simulink model "Wall_Model_Version_1_2"  (R2018a)
settings: Solver=ode3  StartTime=0.0  StopTime=Duration  FixedStep=Ts  RelTol=1e-3  EnableMultiTasking=on
InitFcn:
  | Ts=1;
  | Duration=36000;
  | %% Coefficients of Rs and Cs
  | y1 = 0.5
  | x1 = 0.33;
  | y2 = 0.5;
  | x2 = 0.33;
  | x3 = 0.33;
  | 
  | y3 = 0.5
  | x4 = 0.33;
  | y4 = 0.5;
  | x5 = 0.33;
  | x6 = 0.33;
  | 
  | y5 = 0.5
  | x7 = 0.33;
  | y6 = 0.5;
  | x8 = 0.33;
  | x9 = 0.33;
  | 
  | y7 = 0.5
  | x10 = 0.33;
  | y8 = 0.5;
  | x11 = 0.33;
  | x12= 0.33;
  | 
  | y9 = 0.5
  | x13 = 0.33;
  | y10 = 0.5;
  | x14 = 0.33;
  | x15 = 0.33;
  | 
  | y11 = 0.5
  | x16 = 0.33;
  | y12 = 0.5;
  | x17 = 0.33;
  | x18 = 0.33;
  | 
  | T1_initial_front=28;
  | T2_initial_front=27;
  | 
  | T1_initial_left=28;
  | T2_initial_left=27;
  | 
  | T1_initial_right=28;
  | T2_initial_right=27;
  | 
  | T1_initial_back=28;
  | T2_initial_back=27;
  | 
  | T1_initial_roof=28;
  | T2_initial_roof=27;
  | 
  | T1_initial_floor=28;
  | T2_initial_floor=27;
  | 
  | %% Resistance and Capacitance of front Wall
  | Rth1 = 1/0.8; % Common building brick conductivity = 0.8
  | Cth1 = 1000; % average thermal capcitance
  | 
  | %% Resistance and Capacitance of left Wall
  | Rth2 = 1/0.8; % Common building brick conductivity = 0.8
  | Cth2 = 1000; % average thermal capcitance
  | 
  | %% Resistance and Capacitance of right Wall
  | Rth3 = 1/0.8; % Common building brick conductivity = 0.8
  | Cth3 = 1000; % average thermal capcitance
  | 
  | %% Resistance and Capacitance of back Wall
  | Rth4 = 1/0.8; % Common building brick conductivity = 0.8
  | Cth4 = 1000; % average thermal capcitance
  | 
  | %% Resistance and Capacitance of roof Wall
  | Rth5 = 1/0.8; % Common building brick conductivity = 0.8
  | Cth5 = 1000; % average thermal capcitance
  | 
  | %% Resistance and Capacitance of floor Wall
  | Rth6 = 1/0.8; % Common building brick conductivity = 0.8
  | Cth6 = 1000; % average thermal capcitance
libraries: powerlib x66, simulink x1
settings Model: Creator=elekkr  LastModifiedBy=e0154145
settings DataIOCC: LimitDataPoints=on  SaveFormat=Array
settings OptimizationCC: LifeSpan=inf
settings DebuggingCC: UnconnectedInputMsg=none  UnconnectedOutputMsg=none  UnconnectedLineMsg=none  SFUnexpectedBacktrackingDiag=warning  SFNoUnconditionalDefaultTransitionDiag=warning  SFExecutionAtInitializationDiag=none
settings HardwareCC: ProdBitPerPointer=32  ProdBitPerSizeT=32  ProdBitPerPtrDiffT=32  ProdLargestAtomicFloat=None  ProdIntDivRoundTo=Undefined  ProdEndianess=Unspecified  ProdWordSize=32  ProdHWDeviceType=32-bit Generic
settings ModelReferenceCC: PropagateSignalLabelsOutOfModel=off
settings CodeAppCC: StateflowObjectComments=on
settings GRTTargetCC: TargetLangStandard=C89/C90 (ANSI)  GeneratePreprocessorConditionals=Disable all
settings ConfigComp: CovMetricSettings=dw  CovHtmlReporting=on  CovSaveCumulativeToWorkspaceVar=on  CovSaveSingleToWorkspaceVar=on  CovExternalEMLEnable=off
settings SimscapeCC: SimscapeNormalizeSystem=off

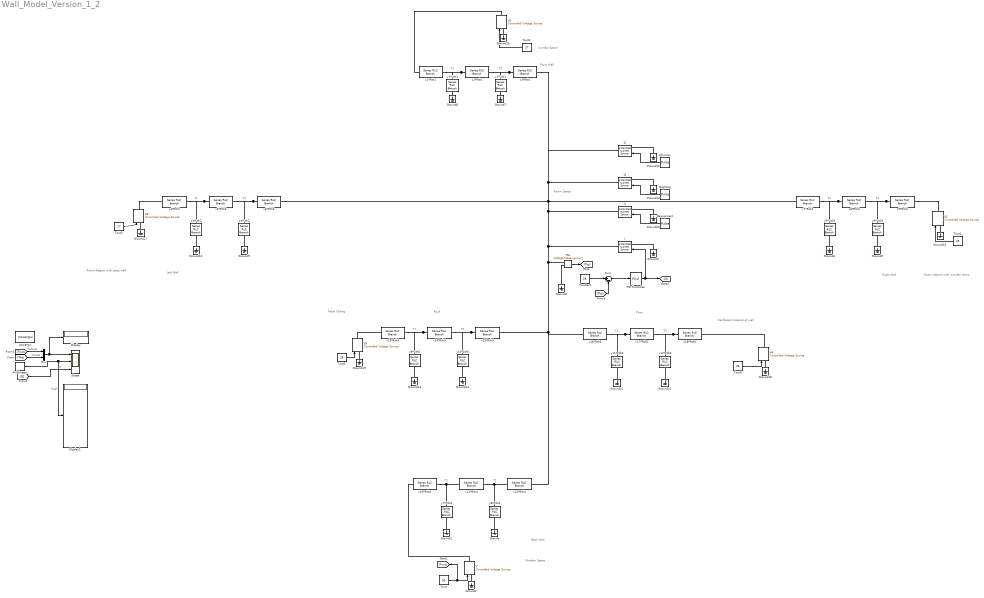
== system Wall_Model_Version_1_2 ==
  note: T1
  note: T2
  note: Back Wall
  note: Room Space
  note: Outdoor Space
  note: T1
  note: T2
  note: T1
  note: T2
  note: T1
  note: T2
  note: T2
  note: T1
  note: T1
  note: T2
  note: Right Wall
  note: Front Wall
  note: Left Wall
  note: Floor
  note: Roof
  note: Room Adjacnt with glass wall
  note: Corridpr Space
  note: Room Adjacnt with wooden doors
  note: Cardboard material of wall
  note: False Ceiling
  Constant : Constant  Value=28
  Display : Display
  Display1 : Display
  Ground{,1..22} (23 alike) : powerlib/Elements/Ground  LConnTagsString=a
  I{,1..3} (4 alike) : powerlib/Electrical Sources/Controlled Current Source  Initialize=on  Source_Type=AC  Amplitude=0  Phase=0  Frequency=0  Measurements=None
  Multimeter : powerlib/Measurements/Multimeter  PhasorSimulation=off  OutputType=Complex  sel=[1 2 3 4 5 6 7 8 9 10 11 12]  L=12  Gain=[1 1 1 1 1 1 1 1 1 1 1 1]  yselected={'Ub: y7*Cth4','Ub: y5*Cth3','Ub: y1*Cth1','Ub: y3*Cth2','Ub: y11*Cth6','Ub: y9*Cth5','Ub: y8*Cth4','Ub: y6*Cth3','Ub: y2*Cth1','Ub: y4*Cth2','Ub: y12*Cth6','Ub: y10*Cth5'};  PSBOutputType=1  PSBequivalent=0  AxesSetting=[0,0.1,-100,100]  Display=0  SavedBlockNames=-11
  Mux : Mux  Inputs=2
  PID Controller : simulink/Continuous/PID Controller  Controller=PI  TimeDomain=Continuous-time  SampleTime=-1  IntegratorMethod=Forward Euler  FilterMethod=Forward Euler  Form=Parallel  UseFilter=on  ControllerParametersSource=internal  P=0  I=7.47908470126143  D=-10.8576065611478  N=0.230769833384862  InitialConditionSource=internal  InitialConditionForIntegrator=25  InitialConditionForFilter=0  ExternalReset=none  LimitOutput=on  UpperSaturationLimit=0  LowerSaturationLimit=-10  LinearizeAsGain=on  AntiWindupMode=none  Kb=1  TrackingMode=off  Kt=1  PParamMin=[]  PParamMax=[]  IParamMin=[]  IParamMax=[]  DParamMin=[]  DParamMax=[]  NParamMin=[]  NParamMax=[]  KbParamMin=[]  KbParamMax=[]  KtParamMin=[]  KtParamMax=[]  POutMin=[]  POutMax=[]  IOutMin=[]  IOutMax=[]  DOutMin=[]  DOutMax=[]  NOutMin=[]  NOutMax=[]  KbOutMin=[]  KbOutMax=[]  KtOutMin=[]  KtOutMax=[]  IntegratorOutMin=[]  IntegratorOutMax=[]  FilterOutMin=[]  FilterOutMax=[]  SumOutMin=[]  SumOutMax=[]  SumI1OutMin=[]  SumI1OutMax=[]  SumI2OutMin=[]  SumI2OutMax=[]  SumI3OutMin=[]  SumI3OutMax=[]  SumDOutMin=[]  SumDOutMax=[]  SaturationOutMin=[]  SaturationOutMax=[]  IntegratorContinuousStateAttributes=''  IntegratorStateMustResolveToSignalObject=off  IntegratorRTWStateStorageClass=Auto  FilterContinuousStateAttributes=''  FilterStateMustResolveToSignalObject=off  FilterRTWStateStorageClass=Auto  DifferentiatorICPrevScaledInput=0  DifferentiatorOutMin=[]  DifferentiatorOutMax=[]  FilterDiffOutCoefMin=[]  FilterDiffOutCoefMax=[]  SumDenOutMin=[]  SumDenOutMax=[]  SumNumOutMin=[]  SumNumOutMax=[]  ReciprocalOutMin=[]  ReciprocalOutMax=[]  DivideOutMin=[]  DivideOutMax=[]  TunerSelectOption=Transfer Function Based (PID Tuner App)
  Qequipment : DiscretePulseGenerator  PulseType=Time based  Period=1e5  PulseWidth=50  PhaseDelay=1e4
  Qhuman : DiscretePulseGenerator  PulseType=Time based  Amplitude=0.5  Period=1e5  PulseWidth=50  PhaseDelay=1e4
  Qlighting : DiscretePulseGenerator  PulseType=Time based  Amplitude=0.75  Period=1e5  PulseWidth=50  PhaseDelay=1e4
  Scope : Scope  NumInputPorts=3
  Sum : Sum  Inputs=|+-
  Tbs : powerlib/Measurements/Voltage Measurement  PhasorSimulation=off  OutputType=Complex  PSBequivalent=0
  Tout : Constant  Value=30
  Tout1 : Constant  Value=25
  Tout2 : Constant  Value=27
  Tout3 : Constant  Value=27
  Tout4 : Constant  Value=26
  Tout5 : Constant  Value=28
  V{,1..5} (6 alike) : powerlib/Electrical Sources/Controlled Voltage Source  Initialize=on  Source_Type=AC  Amplitude=0  Phase=0  Frequency=0  Measurements=None
  powergui : powerlib/powergui  Priority=1  SimulationMode=Discrete  SampleTime=Ts  frequency=60  Iterations=50  frequencyindice=0  Pbase=100e6  ErrMax=1e-4  UnitsV=kV  UnitsW=MW  buscounter=0  FunctionMessages=off  echomessages=off  EnableUseOfTLC=off  CurrentSourceSwitches=off  DisableSnubberDevices=off  DisableRonSwitches=off  DisableVfSwitches=off  DisplayEquations=off  SolverType=Tustin/Backward Euler (TBE)  Interpol=off  ExternalGateDelay=off  methode=off  Ts=100  x0status=blocks  SPID=off  SwTol=0  HookPort=off  RestoreLinks=warning  ResistiveCurrentMeasurement=off  Frange=[0:2:500]  Ylog=off  Xlog=on  ShowGrid=off  save=off  variable=ZData  structure=0  ZoomFFT=off  StartTime=0.0  cycles=1  DisplayStyle=1  fundamental=60  FreqAxis=off  MaxFrequency=1000  frequencyindicesteady=1  RmsSteady=1  display=off
  x1*Rth1 : powerlib/Elements/Series RLC Branch  LConnTagsString=__new0  RConnTagsString=__new0  BranchType=R  Resistance=x1*Rth1  Inductance=1e-3  SetiL0=off  InitialCurrent=0  Capacitance=1e-6  Setx0=off  InitialVoltage=0  Measurements=None
  x10*Rth4 : powerlib/Elements/Series RLC Branch  LConnTagsString=__new0  RConnTagsString=__new0  BranchType=R  Resistance=x10*Rth4  Inductance=1e-3  SetiL0=off  InitialCurrent=0  Capacitance=1e-6  Setx0=off  InitialVoltage=0  Measurements=None
  x11*Rth4 : powerlib/Elements/Series RLC Branch  LConnTagsString=__new0  RConnTagsString=__new0  BranchType=R  Resistance=x11*Rth4  Inductance=1e-3  SetiL0=off  InitialCurrent=0  Capacitance=1e-6  Setx0=off  InitialVoltage=0  Measurements=None
  x12*Rth4 : powerlib/Elements/Series RLC Branch  LConnTagsString=__new0  RConnTagsString=__new0  BranchType=R  Resistance=x12*Rth4  Inductance=1e-3  SetiL0=off  InitialCurrent=0  Capacitance=1e-6  Setx0=off  InitialVoltage=0  Measurements=None
  x13*Rth5 : powerlib/Elements/Series RLC Branch  LConnTagsString=__new0  RConnTagsString=__new0  BranchType=R  Resistance=x13*Rth5  Inductance=1e-3  SetiL0=off  InitialCurrent=0  Capacitance=1e-6  Setx0=off  InitialVoltage=0  Measurements=None
  x14*Rth5 : powerlib/Elements/Series RLC Branch  LConnTagsString=__new0  RConnTagsString=__new0  BranchType=R  Resistance=x14*Rth5  Inductance=1e-3  SetiL0=off  InitialCurrent=0  Capacitance=1e-6  Setx0=off  InitialVoltage=0  Measurements=None
  x15*Rth5 : powerlib/Elements/Series RLC Branch  LConnTagsString=__new0  RConnTagsString=__new0  BranchType=R  Resistance=x15*Rth5  Inductance=1e-3  SetiL0=off  InitialCurrent=0  Capacitance=1e-6  Setx0=off  InitialVoltage=0  Measurements=None
  x16*Rth6 : powerlib/Elements/Series RLC Branch  LConnTagsString=__new0  RConnTagsString=__new0  BranchType=R  Resistance=x16*Rth6  Inductance=1e-3  SetiL0=off  InitialCurrent=0  Capacitance=1e-6  Setx0=off  InitialVoltage=0  Measurements=None
  x17*Rth6 : powerlib/Elements/Series RLC Branch  LConnTagsString=__new0  RConnTagsString=__new0  BranchType=R  Resistance=x17*Rth6  Inductance=1e-3  SetiL0=off  InitialCurrent=0  Capacitance=1e-6  Setx0=off  InitialVoltage=0  Measurements=None
  x18*Rth6 : powerlib/Elements/Series RLC Branch  LConnTagsString=__new0  RConnTagsString=__new0  BranchType=R  Resistance=x18*Rth6  Inductance=1e-3  SetiL0=off  InitialCurrent=0  Capacitance=1e-6  Setx0=off  InitialVoltage=0  Measurements=None
  x2*Rth1 : powerlib/Elements/Series RLC Branch  LConnTagsString=__new0  RConnTagsString=__new0  BranchType=R  Resistance=x2*Rth1  Inductance=1e-3  SetiL0=off  InitialCurrent=0  Capacitance=1e-6  Setx0=off  InitialVoltage=0  Measurements=None
  x3*Rth1 : powerlib/Elements/Series RLC Branch  LConnTagsString=__new0  RConnTagsString=__new0  BranchType=R  Resistance=x3*Rth1  Inductance=1e-3  SetiL0=off  InitialCurrent=0  Capacitance=1e-6  Setx0=off  InitialVoltage=0  Measurements=None
  x4*Rth2 : powerlib/Elements/Series RLC Branch  LConnTagsString=__new0  RConnTagsString=__new0  BranchType=R  Resistance=x4*Rth2  Inductance=1e-3  SetiL0=off  InitialCurrent=0  Capacitance=1e-6  Setx0=off  InitialVoltage=0  Measurements=None
  x5*Rth2 : powerlib/Elements/Series RLC Branch  LConnTagsString=__new0  RConnTagsString=__new0  BranchType=R  Resistance=x5*Rth2  Inductance=1e-3  SetiL0=off  InitialCurrent=0  Capacitance=1e-6  Setx0=off  InitialVoltage=0  Measurements=None
  x6*Rth2 : powerlib/Elements/Series RLC Branch  LConnTagsString=__new0  RConnTagsString=__new0  BranchType=R  Resistance=x6*Rth2  Inductance=1e-3  SetiL0=off  InitialCurrent=0  Capacitance=1e-6  Setx0=off  InitialVoltage=0  Measurements=None
  x7*Rth3 : powerlib/Elements/Series RLC Branch  LConnTagsString=__new0  RConnTagsString=__new0  BranchType=R  Resistance=x7*Rth3  Inductance=1e-3  SetiL0=off  InitialCurrent=0  Capacitance=1e-6  Setx0=off  InitialVoltage=0  Measurements=None
  x8*Rth3 : powerlib/Elements/Series RLC Branch  LConnTagsString=__new0  RConnTagsString=__new0  BranchType=R  Resistance=x8*Rth3  Inductance=1e-3  SetiL0=off  InitialCurrent=0  Capacitance=1e-6  Setx0=off  InitialVoltage=0  Measurements=None
  x9*Rth3 : powerlib/Elements/Series RLC Branch  LConnTagsString=__new0  RConnTagsString=__new0  BranchType=R  Resistance=x9*Rth3  Inductance=1e-3  SetiL0=off  InitialCurrent=0  Capacitance=1e-6  Setx0=off  InitialVoltage=0  Measurements=None
  y1*Cth1 : powerlib/Elements/Series RLC Branch  LConnTagsString=__new0  RConnTagsString=__new0  BranchType=C  Resistance=0  Inductance=1e-3  SetiL0=off  InitialCurrent=0  Capacitance=y1*Cth1  Setx0=on  InitialVoltage=T1_initial_front  Measurements=Branch voltage
  y10*Cth5 : powerlib/Elements/Series RLC Branch  LConnTagsString=__new0  RConnTagsString=__new0  BranchType=C  Resistance=0  Inductance=1e-3  SetiL0=off  InitialCurrent=0  Capacitance=y10*Cth5  Setx0=on  InitialVoltage=T2_initial_roof  Measurements=Branch voltage
  y11*Cth6 : powerlib/Elements/Series RLC Branch  LConnTagsString=__new0  RConnTagsString=__new0  BranchType=C  Resistance=0  Inductance=1e-3  SetiL0=off  InitialCurrent=0  Capacitance=y11*Cth6  Setx0=on  InitialVoltage=T1_initial_floor  Measurements=Branch voltage
  y12*Cth6 : powerlib/Elements/Series RLC Branch  LConnTagsString=__new0  RConnTagsString=__new0  BranchType=C  Resistance=0  Inductance=1e-3  SetiL0=off  InitialCurrent=0  Capacitance=y12*Cth6  Setx0=on  InitialVoltage=T2_initial_floor  Measurements=Branch voltage
  y2*Cth1 : powerlib/Elements/Series RLC Branch  LConnTagsString=__new0  RConnTagsString=__new0  BranchType=C  Resistance=0  Inductance=1e-3  SetiL0=off  InitialCurrent=0  Capacitance=y2*Cth1  Setx0=on  InitialVoltage=T2_initial_front  Measurements=Branch voltage
  y3*Cth2 : powerlib/Elements/Series RLC Branch  LConnTagsString=__new0  RConnTagsString=__new0  BranchType=C  Resistance=0  Inductance=1e-3  SetiL0=off  InitialCurrent=0  Capacitance=y3*Cth2  Setx0=on  InitialVoltage=T1_initial_left  Measurements=Branch voltage
  y4*Cth2 : powerlib/Elements/Series RLC Branch  LConnTagsString=__new0  RConnTagsString=__new0  BranchType=C  Resistance=0  Inductance=1e-3  SetiL0=off  InitialCurrent=0  Capacitance=y4*Cth2  Setx0=on  InitialVoltage=T2_initial_left  Measurements=Branch voltage
  y5*Cth3 : powerlib/Elements/Series RLC Branch  LConnTagsString=__new0  RConnTagsString=__new0  BranchType=C  Resistance=0  Inductance=1e-3  SetiL0=off  InitialCurrent=0  Capacitance=y5*Cth3  Setx0=on  InitialVoltage=T1_initial_right  Measurements=Branch voltage
  y6*Cth3 : powerlib/Elements/Series RLC Branch  LConnTagsString=__new0  RConnTagsString=__new0  BranchType=C  Resistance=0  Inductance=1e-3  SetiL0=off  InitialCurrent=0  Capacitance=y6*Cth3  Setx0=on  InitialVoltage=T2_initial_right  Measurements=Branch voltage
  y7*Cth4 : powerlib/Elements/Series RLC Branch  LConnTagsString=__new0  RConnTagsString=__new0  BranchType=C  Resistance=0  Inductance=1e-3  SetiL0=off  InitialCurrent=0  Capacitance=y7*Cth4  Setx0=on  InitialVoltage=T1_initial_back  Measurements=Branch voltage
  y8*Cth4 : powerlib/Elements/Series RLC Branch  LConnTagsString=__new0  RConnTagsString=__new0  BranchType=C  Resistance=0  Inductance=1e-3  SetiL0=off  InitialCurrent=0  Capacitance=y8*Cth4  Setx0=on  InitialVoltage=T2_initial_back  Measurements=Branch voltage
  y9*Cth5 : powerlib/Elements/Series RLC Branch  LConnTagsString=__new0  RConnTagsString=__new0  BranchType=C  Resistance=0  Inductance=1e-3  SetiL0=off  InitialCurrent=0  Capacitance=y9*Cth5  Setx0=on  InitialVoltage=T1_initial_roof  Measurements=Branch voltage
  wires:
  Tout/1 -> [Tout], V/1
  Tbs/1 -> [Tbs]
  Mux/1 -> Display/1, Scope/1
  [Tbs] -> Mux/2  "Tinside"
  [Tout] -> Mux/1  "Toutside"
  Multimeter/1 -> Display1/1, Scope/2  "Twall"
  [Q] -> Scope/3  "Q"
  Tout1/1 -> V1/1
  Tout2/1 -> V2/1
  Tout3/1 -> V3/1
  Tout4/1 -> V4/1
  Tout5/1 -> V5/1
  Qequipment/1 -> I1/1
  Qhuman/1 -> I2/1
  Qlighting/1 -> I3/1
  PID Controller/1 -> I/1, [Q]
  Sum/1 -> PID Controller/1
  Constant/1 -> Sum/1
  [Tbs] -> Sum/2
  connections:
  x10*Rth4/RConn1 -- y7*Cth4/LConn1 -- x11*Rth4/LConn1
  x11*Rth4/RConn1 -- y8*Cth4/LConn1 -- x12*Rth4/LConn1
  x7*Rth3/LConn1 -- I2/RConn1 -- x3*Rth1/RConn1 -- I3/RConn1 -- x6*Rth2/RConn1 -- I1/RConn1 -- I/RConn1 -- Tbs/LConn1 -- x16*Rth6/LConn1 -- x12*Rth4/RConn1 -- x15*Rth5/RConn1
  Ground/LConn1 -- y8*Cth4/RConn1
  Ground1/LConn1 -- y7*Cth4/RConn1
  V/RConn1 -- x10*Rth4/LConn1
  Ground2/LConn1 -- V/LConn1
  Ground3/LConn1 -- I/LConn1
  Ground4/LConn1 -- Tbs/LConn2
  x9*Rth3/LConn1 -- x8*Rth3/RConn1 -- y6*Cth3/LConn1
  x8*Rth3/LConn1 -- x7*Rth3/RConn1 -- y5*Cth3/LConn1
  Ground5/LConn1 -- y6*Cth3/RConn1
  Ground6/LConn1 -- y5*Cth3/RConn1
  x3*Rth1/LConn1 -- x2*Rth1/RConn1 -- y2*Cth1/LConn1
  x2*Rth1/LConn1 -- x1*Rth1/RConn1 -- y1*Cth1/LConn1
  Ground7/LConn1 -- y2*Cth1/RConn1
  Ground8/LConn1 -- y1*Cth1/RConn1
  x6*Rth2/LConn1 -- x5*Rth2/RConn1 -- y4*Cth2/LConn1
  x5*Rth2/LConn1 -- x4*Rth2/RConn1 -- y3*Cth2/LConn1
  Ground9/LConn1 -- y4*Cth2/RConn1
  Ground10/LConn1 -- y3*Cth2/RConn1
  x17*Rth6/LConn1 -- x16*Rth6/RConn1 -- y11*Cth6/LConn1
  x18*Rth6/LConn1 -- x17*Rth6/RConn1 -- y12*Cth6/LConn1
  Ground11/LConn1 -- y11*Cth6/RConn1
  Ground12/LConn1 -- y12*Cth6/RConn1
  x15*Rth5/LConn1 -- x14*Rth5/RConn1 -- y10*Cth5/LConn1
  x14*Rth5/LConn1 -- x13*Rth5/RConn1 -- y9*Cth5/LConn1
  Ground13/LConn1 -- y9*Cth5/RConn1
  Ground14/LConn1 -- y10*Cth5/RConn1
  Ground15/LConn1 -- V1/LConn1
  x1*Rth1/LConn1 -- V2/RConn1
  Ground16/LConn1 -- V2/LConn1
  x4*Rth2/LConn1 -- V3/RConn1
  Ground17/LConn1 -- V3/LConn1
  Ground18/LConn1 -- V4/LConn1
  x13*Rth5/LConn1 -- V5/RConn1
  Ground19/LConn1 -- V5/LConn1
  Ground20/LConn1 -- I1/LConn1
  Ground21/LConn1 -- I2/LConn1
  Ground22/LConn1 -- I3/LConn1
  x9*Rth3/RConn1 -- V1/RConn1
  V4/RConn1 -- x18*Rth6/RConn1
